simulink model "mcb_pmsm_host_offsetComputation"  (R2025b)
settings: Solver=FixedStepDiscrete  StartTime=0.0  StopTime=inf  RelTol=1e-3  EnableMultiTasking=on
StartFcn:
  | set_param([bdroot '/Serial Communication/Emergency Stop'], 'Value', '1');
values from neighbouring files (symbols this model uses):
  Ts = T_pwm    (= 5e-05)    [mcb_pmsm_foc_f280049C_data.m]    (also in mcb_pmsm_foc_f28335_data.m; mcb_pmsm_foc_qep_f28035_data.m)
undefined symbols (not defined in the file or in its folder): motor
libraries: simulink x4, instrumentseriallib x3, mcbcontrolslib x2, demo_controls x1, mcbpositiondecoderlib x1

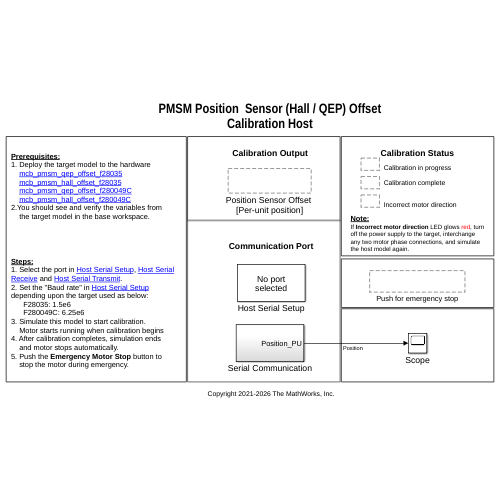
[thumbnail: Simulink's stored preview of the top-level diagram]
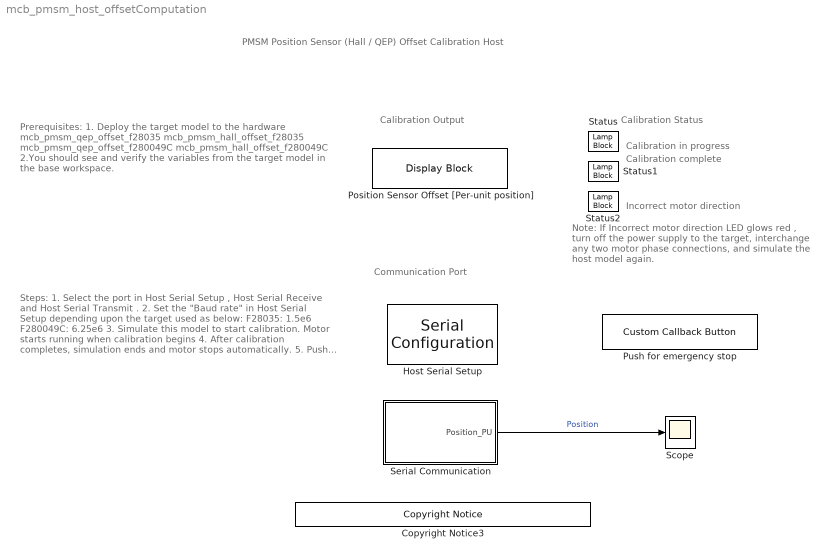
== system mcb_pmsm_host_offsetComputation ==
  note: PMSM Position Sensor (Hall / QEP) Offset Calibration Host
  note: Steps:
      | 1. Select the port in Host Serial Setup , Host Serial Receive and Host Serial Transmit .
      | 2. Set the "Baud rate" in Host Serial Setup depending upon the target used as below:
      | F28035: 1.5e6
      | F280049C: 6.25e6
      | 3. Simulate this model to start calibration.
      | Motor starts running when calibration begins
      | 4. After calibration completes, simulation ends
      | and motor stops automatically.
      | 5. Push the Emergency Motor Stop button to
      | stop the motor during emergency.
  note: Prerequisites:
      | 1. Deploy the target model to the hardware
      | mcb_pmsm_qep_offset_f28035
      | mcb_pmsm_hall_offset_f28035
      | mcb_pmsm_qep_offset_f280049C
      | mcb_pmsm_hall_offset_f280049C
      | 2.You should see and verify the variables from
      | the target model in the base workspace.
  note: Calibration in progress
  note: Calibration complete
  note: Incorrect motor direction
  note: Note:
      | If Incorrect motor direction LED glows red , turn off the power supply to the target, interchange any two motor phase connections, and simulate the host model again.
  note: Calibration Status
  note: Calibration Output
  note: Communication Port
  Copyright Notice3 : demo_controls/Copyright Notice  year=2021  prod=tic2000
  Host Serial Setup : instrumentseriallib/Serial Configuration  Priority=-99  PortSel=<Select a port...>  Port=<Select a port...>  ComPort=<Select a port...>  BaudRate=1.5e6  DataBits=8  Parity=none  StopBits=1  ByteOrder=little-endian  FlowControl=none  Timeout=2  SimulateUsing=Interpreted execution  BlockInModel=on  aMode=5
  Position Sensor Offset [Per-unit position] : DisplayBlock  LabelPosition=Hide  Transparency=1  GridColor=[0.0, 0.0, 1.0]
  Push for emergency stop : CustomCallbackButton  Configuration="{\"components\":[{\"name\":\"BackgroundImageComponent\",\"settings\":{\"image\":{\"size\":[0,0],\"src\":\"default\",\"srcOrientation\":\"Right\"},\"position\":[0,0,1,1]}},{\"name\":\"ButtonStateComponent\",\"settings\":{\"buttonType\":\"momentary\",\"clickFcn\":\"set_param([bdroot '\\/Serial Communication\\/Emergency Stop'], 'Value', '0');\",\"onValue\":1,\"position\":[0,0,1,1],\"pressDelay\":\"500\",\"pressFcn\":\"\",\"repeatInterval\":\"0\",\"states ...(+1858 chars)"  CustomBackgroundColor="{\"color\":[0.9568627451,0.9568627451,0.9568627451],\"show\":true}"
  Scope : Scope
  Serial Communication : Subsystem
  Status : LampBlock  LabelPosition=Hide  DefaultColor=[192.0, 192.0, 192.0]
  Status1 : LampBlock  LabelPosition=Hide  DefaultColor=[192.0, 192.0, 192.0]
  Status2 : LampBlock  LabelPosition=Hide  DefaultColor=[192.0, 192.0, 192.0]
  wires:
  Serial Communication/1(Position_PU) -> Scope/1  "Position"

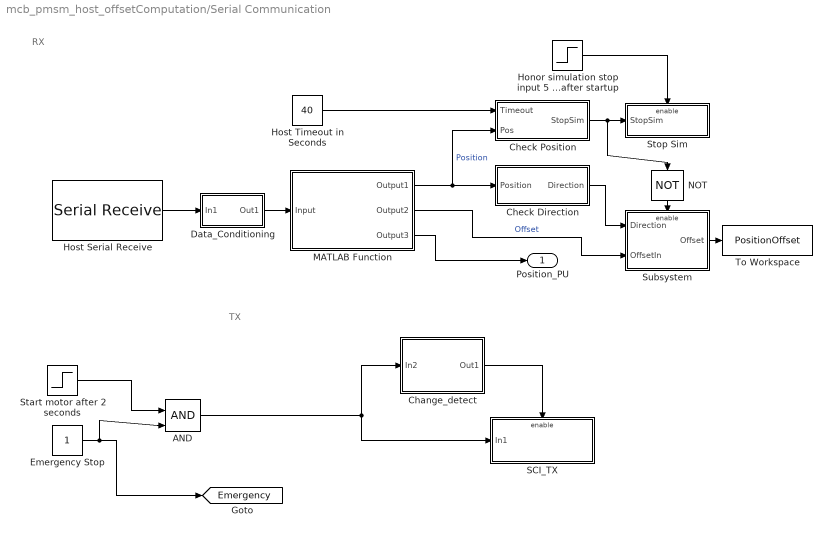
== system mcb_pmsm_host_offsetComputation/Serial Communication ==
  note: RX
  note: TX
  AND : Logic  IconShape=distinctive  AllPortsSameDT=off  OutDataTypeStr=boolean
  Change_detect : Subsystem
  Check Direction : Subsystem
  Check Position : Subsystem
  Data_Conditioning : Subsystem
  Emergency Stop : Constant  OutDataTypeStr=Inherit: Inherit via back propagation
  Honor simulation stop input 5 seconds after startup : Step  Time=5  SampleTime=600*Ts
  Host Serial Receive : instrumentseriallib/Serial Receive  PortSel=<Select a port...>  Port=<Select a port...>  ComPort=<Select a port...>  DataType=uint16  SaveDataType=uint8  ToggleHeader=on  Header='SS'  ToggleDataSize=on  DataSize=[600 2]  ToggleTerminator=on  Terminator=Custom terminator  CustomTerminator='EE'  InputFormat=Row major  EnableBlockingMode=on  ActionDataUnavailable=Output last received value  ActionWhenDataUnavailable=Output last received value  CustomValue=0  SampleTime=600 * Ts  SimulateUsing=Interpreted execution  BlockInModel=on  aMode=5  LibraryInUse=instrumentlib
  Host Timeout in Seconds : Constant  Value=40  OutDataTypeStr=Inherit: Inherit via back propagation
  MATLAB Function : MATLAB Function  TreatAsAtomicUnit=on
  NOT : Logic  Operator=NOT  IconShape=distinctive  AllPortsSameDT=off  OutDataTypeStr=boolean
  SCI_TX : Subsystem  TreatAsAtomicUnit=on
  Start motor after 2 seconds : Step  Time=2  OutDataTypeStr=single  SampleTime=Ts*600
  Stop Sim : Subsystem
  Subsystem : Subsystem
  To Workspace : ToWorkspace  VariableName=PositionOffset  SampleTime=-1
  Position_PU : Outport
  tag scope: Emergency=global
  wires:
  MATLAB Function/3(Output3) -> Position_PU/1
  MATLAB Function/2(Output2) -> Subsystem/2(OffsetIn)  "Offset"
  Host Serial Receive/1 -> Data_Conditioning/1(In1)
  MATLAB Function/1(Output1) -> Check Position/2(Pos), Check Direction/1(Position)  "Position"
  Data_Conditioning/1(Out1) -> MATLAB Function/1(Input)
  AND/1 -> SCI_TX/1(In1), Change_detect/1(In2)
  Change_detect/1(Out1) -> SCI_TX/Enable
  Honor simulation stop input 5 seconds after startup/1 -> Stop Sim/Enable
  Check Position/1(StopSim) -> NOT/1, Stop Sim/1(StopSim)
  Check Direction/1(Direction) -> Subsystem/1(Direction)
  NOT/1 -> Subsystem/Enable
  Subsystem/1(Offset) -> To Workspace/1
  Emergency Stop/1 -> [Emergency], AND/2
  Start motor after 2 seconds/1 -> AND/1
  Host Timeout in Seconds/1 -> Check Position/1(Timeout)

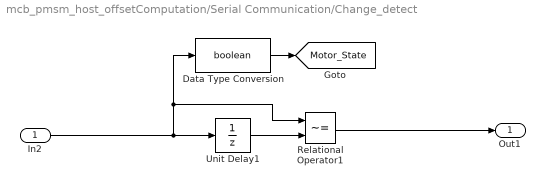
== system mcb_pmsm_host_offsetComputation/Serial Communication/Change_detect ==
  In2 : Inport
  Data Type Conversion : DataTypeConversion  OutDataTypeStr=boolean  RndMeth=Simplest  SaturateOnIntegerOverflow=off
  Relational Operator1 : RelationalOperator  Operator=~=  OutDataTypeStr=boolean  InputSameDT=off
  Unit Delay1 : UnitDelay  SampleTime=-1  HasFrameUpgradeWarning=on
  Out1 : Outport  VectorParamsAs1DForOutWhenUnconnected=off
  tag scope: Motor_State=global
  wires:
  In2/1 -> Data Type Conversion/1, Relational Operator1/1, Unit Delay1/1
  Unit Delay1/1 -> Relational Operator1/2
  Relational Operator1/1 -> Out1/1
  Data Type Conversion/1 -> [Motor_State]

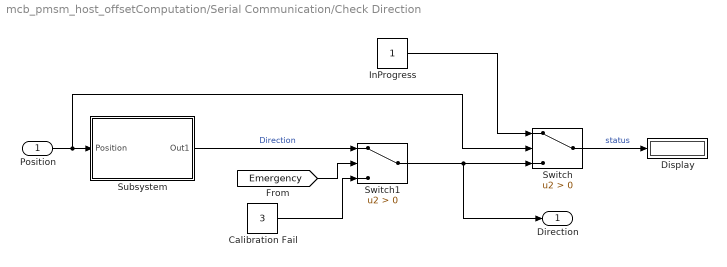
== system mcb_pmsm_host_offsetComputation/Serial Communication/Check Direction ==
  Position : Inport
  Calibration Fail : Constant  Value=3  OutDataTypeStr=uint16
  Display : Display
  InProgress : Constant  OutDataTypeStr=uint16
  Subsystem : Subsystem
  Switch : Switch  Criteria=u2 > Threshold  SaturateOnIntegerOverflow=off  InputSameDT=off
  Switch1 : Switch  Criteria=u2 > Threshold  SaturateOnIntegerOverflow=off  InputSameDT=off
  Direction : Outport
  wires:
  InProgress/1 -> Switch/1
  Position/1 -> Switch/2, Subsystem/1(Position)
  Subsystem/1(Out1) -> Switch1/1  "Direction"
  [Emergency] -> Switch1/2
  Calibration Fail/1 -> Switch1/3
  Switch1/1 -> Direction/1, Switch/3
  Switch/1 -> Display/1  "status"

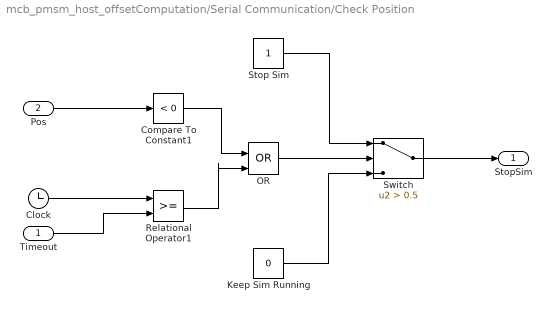
== system mcb_pmsm_host_offsetComputation/Serial Communication/Check Position ==
  Timeout : Inport
  Pos : Inport  Port=2
  Clock : Clock
  Compare To Constant1 : simulink/Logic and Bit Operations/Compare To Constant  relop=<  const=0  OutDataTypeStr=boolean
  Keep Sim Running : Constant  Value=0  OutDataTypeStr=Inherit: Inherit via back propagation
  OR : Logic  Operator=OR  IconShape=distinctive  AllPortsSameDT=off  OutDataTypeStr=boolean
  Relational Operator1 : RelationalOperator  OutDataTypeStr=boolean  RndMeth=Simplest  InputSameDT=off
  Stop Sim : Constant  OutDataTypeStr=Inherit: Inherit via back propagation
  Switch : Switch  Criteria=u2 > Threshold  Threshold=0.5  SaturateOnIntegerOverflow=off  InputSameDT=off
  StopSim : Outport
  wires:
  Pos/1 -> Compare To Constant1/1
  Switch/1 -> StopSim/1
  Clock/1 -> Relational Operator1/1
  Compare To Constant1/1 -> OR/1
  Relational Operator1/1 -> OR/2
  OR/1 -> Switch/2
  Stop Sim/1 -> Switch/1
  Keep Sim Running/1 -> Switch/3
  Timeout/1 -> Relational Operator1/2

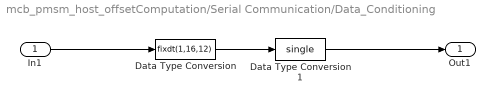
== system mcb_pmsm_host_offsetComputation/Serial Communication/Data_Conditioning ==
  In1 : Inport
  Data Type Conversion : DataTypeConversion  OutDataTypeStr=fixdt(1,16,12)  ConvertRealWorld=Stored Integer (SI)  RndMeth=Simplest  SaturateOnIntegerOverflow=off
  Data Type Conversion1 : DataTypeConversion  OutDataTypeStr=single  SaturateOnIntegerOverflow=off  RndMeth=Floor
  Out1 : Outport  VectorParamsAs1DForOutWhenUnconnected=off
  wires:
  Data Type Conversion1/1 -> Out1/1
  In1/1 -> Data Type Conversion/1
  Data Type Conversion/1 -> Data Type Conversion1/1

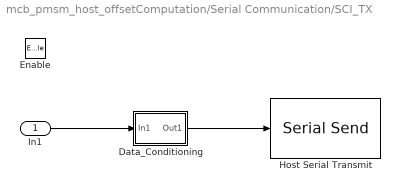
== system mcb_pmsm_host_offsetComputation/Serial Communication/SCI_TX ==
  In1 : Inport
  Enable : EnablePort
  Data_Conditioning : Subsystem
  Host Serial Transmit : instrumentseriallib/Serial Send  PortSel=<Select a port...>  Port=<Select a port...>  ComPort=<Select a port...>  Header=[]  Terminator=<none>  CustomTerminator=[]  EnableBlockingMode=off  SimulateUsing=Interpreted execution  BlockInModel=on  aMode=5
  wires:
  In1/1 -> Data_Conditioning/1(In1)
  Data_Conditioning/1(Out1) -> Host Serial Transmit/1

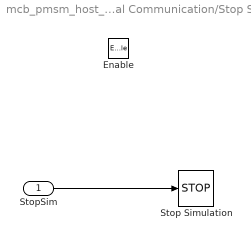
== system mcb_pmsm_host_offsetComputation/Serial Communication/Stop Sim ==
  StopSim : Inport
  Enable : EnablePort
  Stop Simulation : Stop
  wires:
  StopSim/1 -> Stop Simulation/1

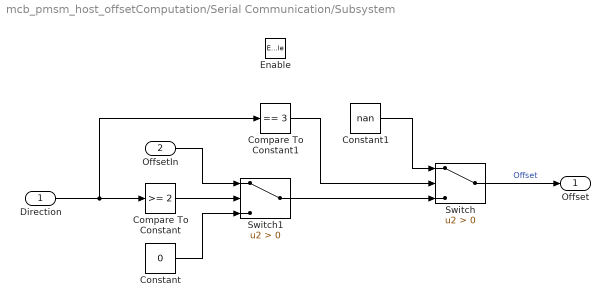
== system mcb_pmsm_host_offsetComputation/Serial Communication/Subsystem ==
  Direction : Inport
  OffsetIn : Inport  Port=2
  Enable : EnablePort
  Compare To Constant : simulink/Logic and Bit Operations/Compare To Constant  relop=>=  const=2  OutDataTypeStr=boolean
  Compare To Constant1 : simulink/Logic and Bit Operations/Compare To Constant  relop===  const=3  OutDataTypeStr=boolean
  Constant : Constant  Value=0  OutDataTypeStr=Inherit: Inherit via back propagation
  Constant1 : Constant  Value=nan  OutDataTypeStr=Inherit: Inherit via back propagation
  Switch : Switch  Criteria=u2 > Threshold  SaturateOnIntegerOverflow=off  InputSameDT=off
  Switch1 : Switch  Criteria=u2 > Threshold  SaturateOnIntegerOverflow=off  InputSameDT=off
  Offset : Outport
  wires:
  Switch/1 -> Offset/1  "Offset"
  Direction/1 -> Compare To Constant1/1, Compare To Constant/1
  Constant/1 -> Switch1/3
  Compare To Constant/1 -> Switch1/2
  OffsetIn/1 -> Switch1/1
  Constant1/1 -> Switch/1
  Compare To Constant1/1 -> Switch/2
  Switch1/1 -> Switch/3

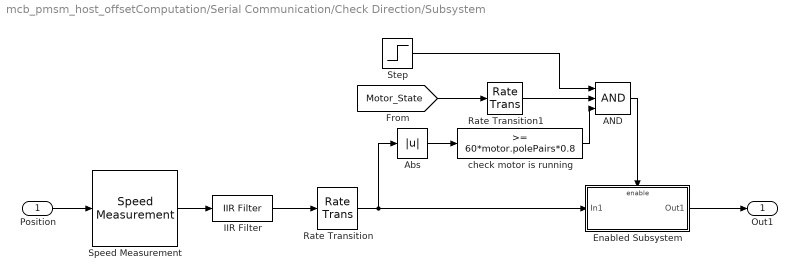
== system mcb_pmsm_host_offsetComputation/Serial Communication/Check Direction/Subsystem ==
  Position : Inport
  AND : Logic  Inputs=3  IconShape=distinctive  AllPortsSameDT=off  OutDataTypeStr=boolean
  Abs : Abs  SaturateOnIntegerOverflow=off
  Enabled Subsystem : Subsystem  TreatAsAtomicUnit=on
  IIR Filter : mcbcontrolslib/IIR Filter  VariantControl=Low Pass Filter  VariantSelect=Low-pass  FilterConstantInputType=Specify via dialog  Filter_constant=0.01  InitialOutput=Specify via dialog  InitialOutputValue=0  ExternalReset=none  advancedSettings=off  Ts=50e-6  cutOff_freq=32.1525
  Rate Transition : RateTransition
  Rate Transition1 : RateTransition
  Speed Measurement : mcbpositiondecoderlib/Speed Measurement  DiscreteStepInput=off  LastDiscreteStepInput=off  PositionUnit=Per unit  PositionScalingDatatype=uint32  SpeedCalculationMode=Maximum application speed  TempSpeedCalculationMode=Time interval for speed calculation  SampleTimeAsync=Ts*600  MaximumApplicationSpeed=4000  SpeedResolution=5e-6  DelayLength=1  MaximumMeasurableSpeed=0.16484  MeasurableSpeedResolution=7.6757e-11  SpeedUnit=RPM  TempSpeedUnit=RPM  PerUnitSpeed=1000  SpeedDataType=single
  Step : Step  Time=5  SampleTime=600*Ts
  check motor is running : simulink/Logic and Bit Operations/Compare To Constant  relop=>=  const=60*motor.polePairs*0.8  OutDataTypeStr=boolean
  Out1 : Outport
  wires:
  Rate Transition/1 -> Enabled Subsystem/1(In1), Abs/1
  Rate Transition1/1 -> AND/2
  Abs/1 -> check motor is running/1
  Position/1 -> Speed Measurement/1
  [Motor_State] -> Rate Transition1/1
  check motor is running/1 -> AND/3
  IIR Filter/1 -> Rate Transition/1
  AND/1 -> Enabled Subsystem/Enable
  Speed Measurement/1 -> IIR Filter/1
  Enabled Subsystem/1(Out1) -> Out1/1
  Step/1 -> AND/1

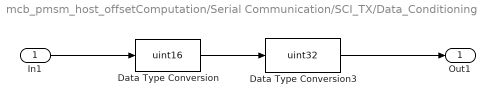
== system mcb_pmsm_host_offsetComputation/Serial Communication/SCI_TX/Data_Conditioning ==
  In1 : Inport
  Data Type Conversion : DataTypeConversion  OutDataTypeStr=uint16  RndMeth=Simplest  SaturateOnIntegerOverflow=off
  Data Type Conversion3 : DataTypeConversion  OutDataTypeStr=uint32  ConvertRealWorld=Stored Integer (SI)  RndMeth=Simplest  SaturateOnIntegerOverflow=off
  Out1 : Outport  VectorParamsAs1DForOutWhenUnconnected=off
  wires:
  Data Type Conversion3/1 -> Out1/1
  Data Type Conversion/1 -> Data Type Conversion3/1
  In1/1 -> Data Type Conversion/1

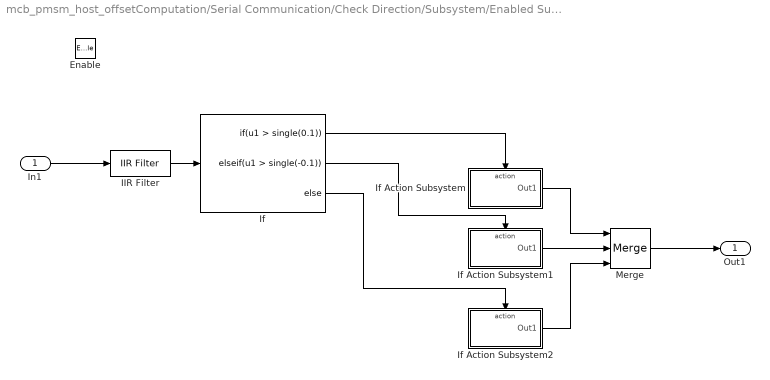
== system mcb_pmsm_host_offsetComputation/Serial Communication/Check Direction/Subsystem/Enabled Subsystem ==
  In1 : Inport
  Enable : EnablePort
  IIR Filter : mcbcontrolslib/IIR Filter  VariantControl=Low Pass Filter  VariantSelect=Low-pass  FilterConstantInputType=Specify via dialog  Filter_constant=0.001  InitialOutput=Specify via dialog  InitialOutputValue=0  ExternalReset=none  advancedSettings=off  Ts=50e-6  cutOff_freq=3.1863
  If : If  IfExpression=u1 > single(0.1)  ElseIfExpressions=u1 > single(-0.1)
  If Action Subsystem : Subsystem  TreatAsAtomicUnit=on
  If Action Subsystem1 : Subsystem  TreatAsAtomicUnit=on
  If Action Subsystem2 : Subsystem  TreatAsAtomicUnit=on
  Merge : Merge  Inputs=3
  Out1 : Outport
  wires:
  In1/1 -> IIR Filter/1
  If/1 -> If Action Subsystem/Action
  If/2 -> If Action Subsystem1/Action
  If/3 -> If Action Subsystem2/Action
  If Action Subsystem/1(Out1) -> Merge/1
  If Action Subsystem1/1(Out1) -> Merge/2
  If Action Subsystem2/1(Out1) -> Merge/3
  IIR Filter/1 -> If/1
  Merge/1 -> Out1/1

== system mcb_pmsm_host_offsetComputation/Serial Communication/Check Direction/Subsystem/Enabled Subsystem/If Action Subsystem ==
  Action Port : ActionPort  ActionPortLabel=if(u1 > single(0.1))
  Motor rotating in correct direction : Constant  Value=2  OutDataTypeStr=uint16
  Out1 : Outport
  wires:
  Motor rotating in correct direction/1 -> Out1/1

== system mcb_pmsm_host_offsetComputation/Serial Communication/Check Direction/Subsystem/Enabled Subsystem/If Action Subsystem1 ==
  Action Port : ActionPort  ActionPortLabel=elseif(u1 > single(-0.1))
  Motor not rotating : Constant  Value=0  OutDataTypeStr=uint16
  Out1 : Outport
  wires:
  Motor not rotating/1 -> Out1/1

== system mcb_pmsm_host_offsetComputation/Serial Communication/Check Direction/Subsystem/Enabled Subsystem/If Action Subsystem2 ==
  Action Port : ActionPort  ActionPortLabel=else
  Motor rotating in wrong direction : Constant  Value=3  OutDataTypeStr=uint16
  Out1 : Outport
  wires:
  Motor rotating in wrong direction/1 -> Out1/1

== matlab function mcb_pmsm_host_offsetComputation/Serial Communication/MATLAB Function ==
function [Output1, Output2, Output3] = unBuf(Input)

selSignal= Input(:, 1);
Output1 = selSignal(1,1);
selSignal = Input(:, 2);
Output2 = selSignal(1,1);
Output3 = Input(:,1);
end
